simulink model "Glide_flare"  (R2020a)
settings: Solver=VariableStepAuto  StartTime=0.0  StopTime=300  RelTol=1e-3
values from neighbouring files (symbols this model uses):
  A_reduced = A_lo([3,7,8,5,11],[3,7,8,5,11])    [landing.m]
  B_reduced = A_lo([3,7,8,5,11], [13,14])    [landing.m]
  C_reduced = C_lo([3,7,8,5,11],[3,7,8,5,11])    [landing.m]
  D_reduced = D_lo([3,7,8,5,11], [1,2])    [landing.m]
  elevator = -0.09    [FindF16Dynamics.m]    (also in runF16Sim.m; runLINF16sim.m)
  thrust = 5000    [FindF16Dynamics.m]    (also in landing.m = 2826.8165; runF16Sim.m; runLINF16sim.m = 0)
undefined symbols (not defined in the file or in its folder): magnitude
libraries: simulink_extras x5
settings Model: Creator=sarka  LastModifiedBy=sarka

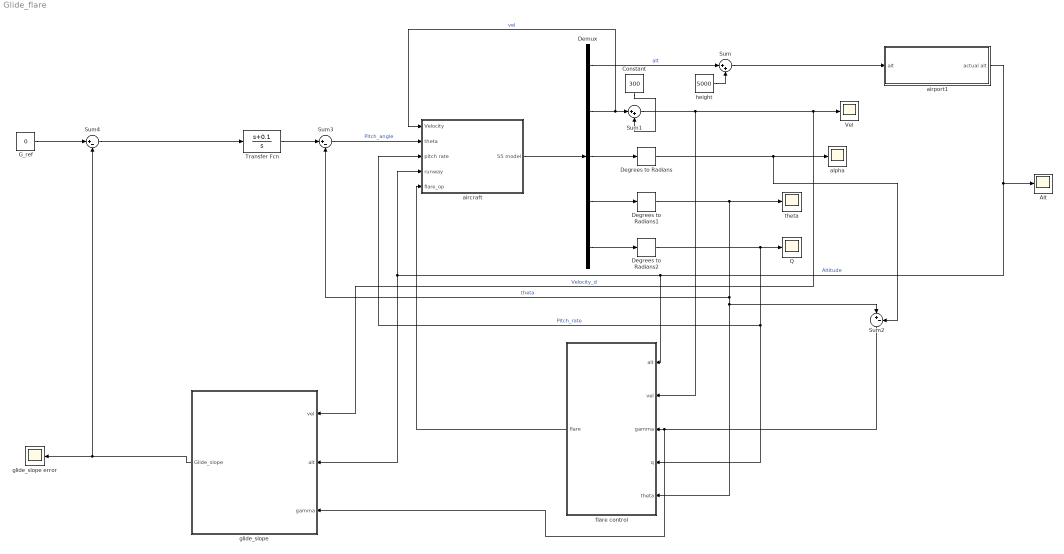
== system Glide_flare ==
  Alt : Scope
  Constant : Constant  Value=300
  Degrees to Radians : simulink_extras/Transformations/Degrees to Radians
  Degrees to Radians1 : simulink_extras/Transformations/Degrees to Radians
  Degrees to Radians2 : simulink_extras/Transformations/Degrees to Radians
  Demux : Demux  Outputs=5
  G_ref : Constant  Value=0
  Q : Scope
  Sum : Sum  Inputs=|++
  Sum1 : Sum  Inputs=|++
  Sum2 : Sum  Inputs=|+-
  Sum3 : Sum  Inputs=|+-
  Sum4 : Sum  Inputs=|+-
  Transfer Fcn : TransferFcn  Numerator=[1 0.1]  Denominator=[1 0]
  Vel : Scope
  aircraft : Subsystem
  airport1 : Subsystem
  alpha : Scope
  flare control : Subsystem
  glide_slope : Subsystem
  glide_slope error : Scope
  height : Constant  Value=5000
  theta : Scope
  wires:
  Degrees to Radians2/1 -> Q/1, aircraft/3(pitch rate), flare control/4(q)  "Pitch_rate"
  Sum/1 -> airport1/1(alt)
  Demux/2 -> aircraft/1(Velocity), Sum1/1  "vel"
  Demux/5 -> Degrees to Radians2/1
  Demux/4 -> Degrees to Radians1/1
  height/1 -> Sum/2
  Demux/1 -> Sum/1  "alt"
  Constant/1 -> Sum1/2
  Degrees to Radians/1 -> alpha/1, Sum2/2
  Sum1/1 -> glide_slope/1(vel), Vel/1, flare control/2(vel)  "Velocity_d"
  aircraft/1(SS model) -> Demux/1
  Demux/3 -> Degrees to Radians/1
  Degrees to Radians1/1 -> theta/1, Sum3/2, Sum2/1, flare control/5(theta)  "theta"
  airport1/1(actual alt) -> Alt/1, flare control/1(alt), glide_slope/2(alt), aircraft/4(runway)  "Altitude"
  flare control/1(flare) -> aircraft/5(flare_op)
  Sum2/1 -> glide_slope/3(gamma), flare control/3(gamma)
  Sum3/1 -> aircraft/2(theta)  "Pitch_angle"
  Transfer Fcn/1 -> Sum3/1
  G_ref/1 -> Sum4/1
  glide_slope/1(Glide_slope) -> glide_slope error/1, Sum4/2
  Sum4/1 -> Transfer Fcn/1

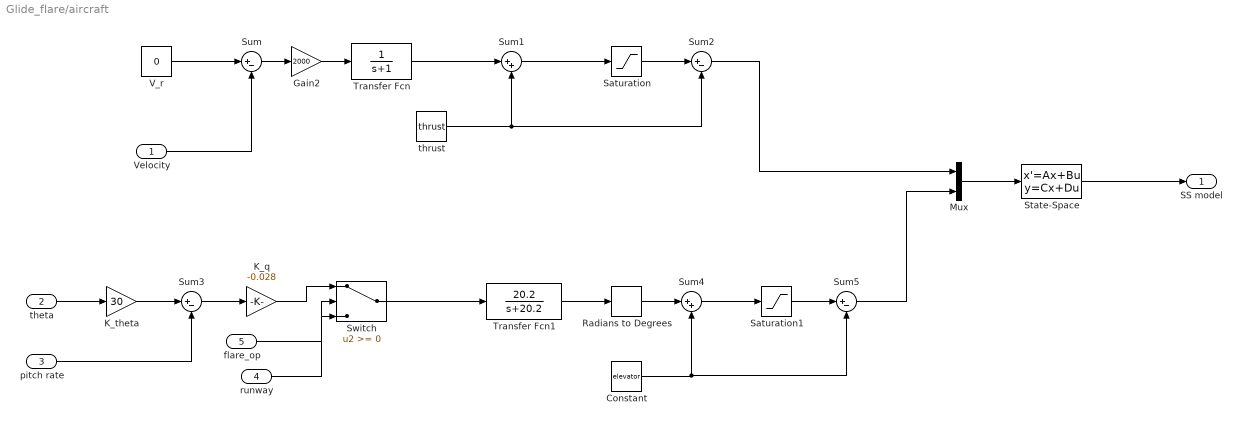
== system Glide_flare/aircraft ==
  Velocity : Inport
  theta : Inport  Port=2
  pitch rate : Inport  Port=3
  runway : Inport  Port=4
  flare_op : Inport  Port=5
  Constant : Constant  Value=elevator
  Gain2 : Gain  Gain=2000
  K_q : Gain  Gain=-0.028
  K_theta : Gain  Gain=30
  Mux : Mux  Inputs=2
  Radians to Degrees : simulink_extras/Transformations/Radians to Degrees
  Saturation : Saturate  UpperLimit=19000  LowerLimit=1000
  Saturation1 : Saturate  UpperLimit=25  LowerLimit=-25
  State-Space : StateSpace  A=A_reduced  B=B_reduced  C=C_reduced  D=D_reduced  InitialCondition=0
  Sum{,2..3,5} (4 alike) : Sum  Inputs=|+-
  Sum1 : Sum  Inputs=|++
  Sum4 : Sum  Inputs=|++
  Switch : Switch
  Transfer Fcn : TransferFcn  Denominator=[1 1]
  Transfer Fcn1 : TransferFcn  Numerator=[20.2]  Denominator=[1 20.2]
  V_r : Constant  Value=0
  thrust : Constant  Value=thrust
  SS model : Outport
  wires:
  K_q/1 -> Switch/1
  Sum/1 -> Gain2/1
  Radians to Degrees/1 -> Sum4/1
  Mux/1 -> State-Space/1
  Sum1/1 -> Saturation/1
  Switch/1 -> Transfer Fcn1/1
  State-Space/1 -> SS model/1
  Transfer Fcn/1 -> Sum1/1
  Sum4/1 -> Saturation1/1
  Transfer Fcn1/1 -> Radians to Degrees/1
  Saturation/1 -> Sum2/1
  runway/1 -> Switch/3
  Sum2/1 -> Mux/1
  theta/1 -> K_theta/1
  Constant/1 -> Sum5/2, Sum4/2
  Sum5/1 -> Mux/2
  thrust/1 -> Sum2/2, Sum1/2
  flare_op/1 -> Switch/2
  Saturation1/1 -> Sum5/1
  pitch rate/1 -> Sum3/2
  V_r/1 -> Sum/1
  Sum3/1 -> K_q/1
  K_theta/1 -> Sum3/1
  Velocity/1 -> Sum/2
  Gain2/1 -> Transfer Fcn/1

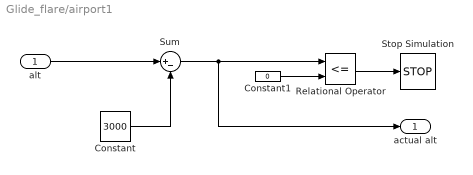
== system Glide_flare/airport1 ==
  alt : Inport
  Constant : Constant  Value=3000
  Constant1 : Constant  Value=0
  Relational Operator : RelationalOperator  Operator=<=  OutDataTypeStr=boolean  RndMeth=Simplest
  Stop Simulation : Stop
  Sum : Sum  Inputs=|+-
  actual alt : Outport
  wires:
  alt/1 -> Sum/1
  Constant/1 -> Sum/2
  Sum/1 -> actual alt/1, Relational Operator/1
  Constant1/1 -> Relational Operator/2
  Relational Operator/1 -> Stop Simulation/1

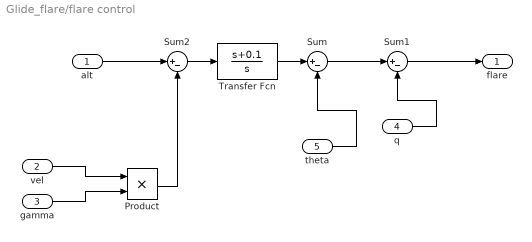
== system Glide_flare/flare control ==
  alt : Inport
  vel : Inport  Port=2
  gamma : Inport  Port=3
  q : Inport  Port=4
  theta : Inport  Port=5
  Product : Product
  Sum : Sum  Inputs=|+-
  Sum1 : Sum  Inputs=|+-
  Sum2 : Sum  Inputs=|+-
  Transfer Fcn : TransferFcn  Numerator=[1 0.1]  Denominator=[1 0]
  flare : Outport
  wires:
  q/1 -> Sum1/2
  Product/1 -> Sum2/2
  Sum/1 -> Sum1/1
  Transfer Fcn/1 -> Sum/1
  alt/1 -> Sum2/1
  vel/1 -> Product/1
  Sum2/1 -> Transfer Fcn/1
  theta/1 -> Sum/2
  Sum1/1 -> flare/1
  gamma/1 -> Product/2

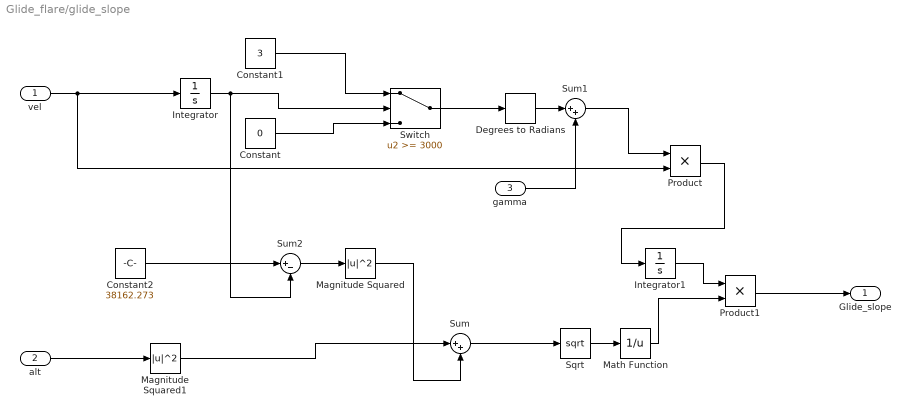
== system Glide_flare/glide_slope ==
  vel : Inport
  alt : Inport  Port=2
  gamma : Inport  Port=3
  Constant : Constant  Value=0
  Constant1 : Constant  Value=3
  Constant2 : Constant  Value=38162.273
  Degrees to Radians : simulink_extras/Transformations/Degrees to Radians
  Integrator : Integrator
  Integrator1 : Integrator
  Magnitude Squared : Math  Operator=magnitude^2  SaturateOnIntegerOverflow=on
  Magnitude Squared1 : Math  Operator=magnitude^2  SaturateOnIntegerOverflow=on
  Math Function : Math  Operator=reciprocal  SignedPower=on  RndMeth=Zero  SaturateOnIntegerOverflow=on
  Product : Product
  Product1 : Product
  Sqrt : Sqrt  SaturateOnIntegerOverflow=on
  Sum : Sum  Inputs=|++
  Sum1 : Sum  Inputs=|++
  Sum2 : Sum  Inputs=|+-
  Switch : Switch  Threshold=3000
  Glide_slope : Outport
  wires:
  vel/1 -> Product/2, Integrator/1
  alt/1 -> Magnitude Squared1/1
  Constant/1 -> Switch/3
  Constant1/1 -> Switch/1
  Integrator/1 -> Sum2/2, Switch/2
  Switch/1 -> Degrees to Radians/1
  Magnitude Squared1/1 -> Sum/1
  Degrees to Radians/1 -> Sum1/1
  gamma/1 -> Sum1/2
  Constant2/1 -> Sum2/1
  Sum2/1 -> Magnitude Squared/1
  Magnitude Squared/1 -> Sum/2
  Sum/1 -> Sqrt/1
  Sqrt/1 -> Math Function/1
  Sum1/1 -> Product/1
  Product/1 -> Integrator1/1
  Integrator1/1 -> Product1/1
  Product1/1 -> Glide_slope/1
  Math Function/1 -> Product1/2
